simulink model "gantryModel"  (R2025b)
settings: Solver=ode4  StartTime=0.0  StopTime=50  FixedStep=0.01  RelTol=1e-3
values from neighbouring files (symbols this model uses):
  Kda = p(3)    [costFun.m]    (also in plots_tuning.m = gains.Kda(id_gain); tuning.m = Kda(valid))
  Kpa = p(2)    [costFun.m]    (also in plots_tuning.m = gains.Kpa(id_gain); tuning.m = Kpa(valid))
  Kpx = p(1)    [costFun.m]    (also in plots_tuning.m = gains.Kpx(id_gain); tuning.m = Kpx(valid))
libraries: simulink x3, SignalEditorBlockLib x2
settings Model: Creator=David  LastModifiedBy=David

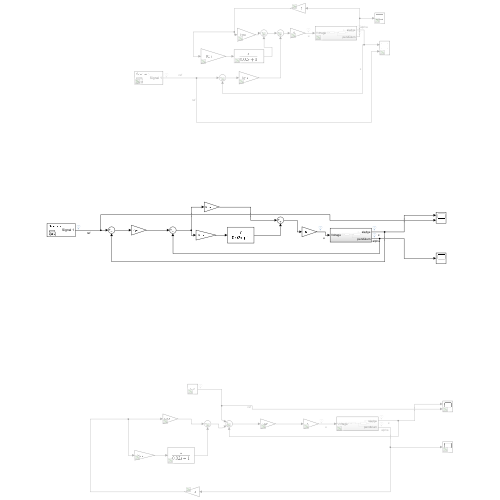
[thumbnail: Simulink's stored preview of the top-level diagram]
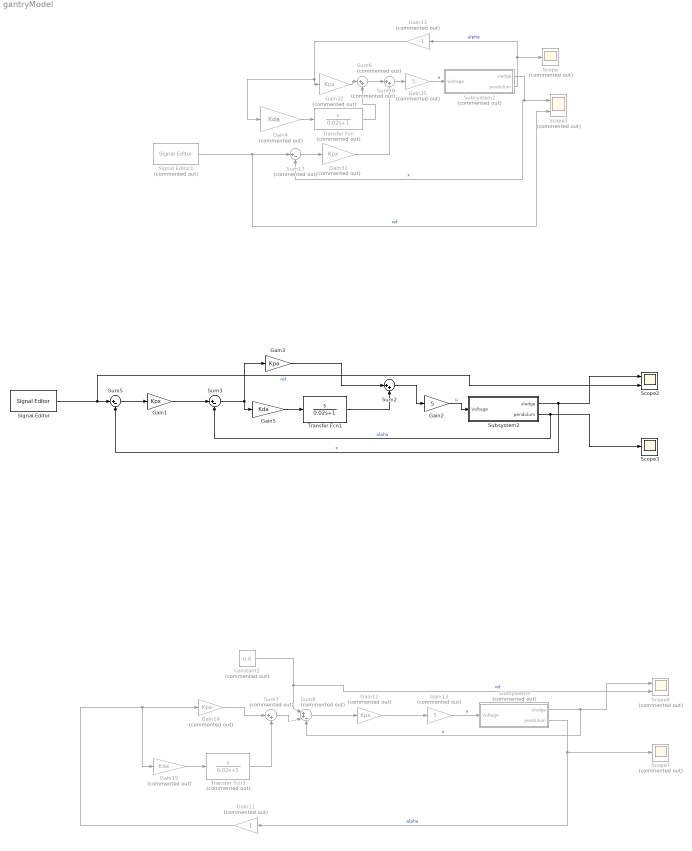
== system gantryModel ==
  Constant2 : Constant  Commented=on  Value=0.8
  Gain1 : Gain  Gain=Kpx
  Gain11 : Gain  Commented=on  Gain=-1
  Gain12 : Gain  Commented=on  Gain=Kpx
  Gain13 : Gain  Commented=on  Gain=5
  Gain14 : Gain  Commented=on  Gain=Kpa
  Gain15 : Gain  Commented=on  Gain=Kda
  Gain2 : Gain  Gain=5
  Gain3 : Gain  Gain=Kpa
  Gain31 : Gain  Commented=on  Gain=Kpx
  Gain32 : Gain  Commented=on  Gain=Kpa
  Gain33 : Gain  Commented=on  Gain=-1
  Gain35 : Gain  Commented=on  Gain=5
  Gain4 : Gain  Commented=on  Gain=Kda
  Gain5 : Gain  Gain=Kda
  Scope : Scope  Commented=on
      settings: ActiveDisplayYMinimum=-4.994410671179125  ActiveDisplayYMaximum=9.4101458764359265
  Scope1 : Scope  Commented=on  NumInputPorts=2
      settings: ActiveDisplayYMinimum=-0.10066051222345068  ActiveDisplayYMaximum=0.90352410472833355
  Scope2 : Scope  NumInputPorts=2
      settings: ActiveDisplayYMinimum=-0.10009126772329788  ActiveDisplayYMaximum=0.90001014085814424  DataLoggingVariableName=ScopeData2
  Scope3 : Scope
      settings: ActiveDisplayYMinimum=-2.552281253947331  ActiveDisplayYMaximum=9.1716981948412979  DataLoggingVariableName=ScopeData3
  Scope6 : Scope  Commented=on  NumInputPorts=2
      settings: ActiveDisplayYMinimum=-0.10533097265407888  ActiveDisplayYMaximum=0.94454271480208  DataLoggingVariableName=ScopeData6
  Scope7 : Scope  Commented=on
      settings: ActiveDisplayYMinimum=-4.9897184342824046  ActiveDisplayYMaximum=9.4373460456385061  DataLoggingVariableName=ScopeData7
  Signal Editor : SignalEditorBlockLib/Signal Editor  FileName=input_tuning.mat  ActiveScenario=Scenario  ActiveSignal=Signal 1  IsBus=off  OutputBusObjectStr=Bus: BusObject  SampleTime=0  ZeroCross=off  OutputAfterFinalValue=Setting to zero  Unit=inherit  PreserveSignalName=on  ApplySigPropsToAllScenarios=on  ApplySigPropsToAllSignals=off  SignalPropertySource=Dialog parameters
  Signal Editor1 : SignalEditorBlockLib/Signal Editor  Commented=on  FileName=input_tuning.mat  ActiveScenario=Scenario  ActiveSignal=Signal 1  IsBus=off  OutputBusObjectStr=Bus: BusObject  SampleTime=0  ZeroCross=off  OutputAfterFinalValue=Setting to zero  Unit=inherit  PreserveSignalName=on  ApplySigPropsToAllScenarios=on  ApplySigPropsToAllSignals=off  SignalPropertySource=Dialog parameters
  Subsystem1 : Subsystem  Commented=on
  Subsystem2 : Subsystem
  Subsystem4 : Subsystem  Commented=on
  Sum16 : Sum  Commented=on  Inputs=|++
  Sum17 : Sum  Commented=on  Inputs=|+-
  Sum2 : Sum  Inputs=|++
  Sum3 : Sum  Inputs=|+-
  Sum5 : Sum  Inputs=|+-
  Sum6 : Sum  Commented=on  Inputs=|++
  Sum7 : Sum  Commented=on  Inputs=|++
  Sum8 : Sum  Commented=on  Inputs=|++-
  Transfer Fcn : TransferFcn  Commented=on  Numerator=[1 0]  Denominator=[0.02 1]
  Transfer Fcn1 : TransferFcn  Numerator=[1 0]  Denominator=[0.02 1]
  Transfer Fcn3 : TransferFcn  Commented=on  Numerator=[1 0]  Denominator=[0.02 1]
  wires:
  Signal Editor1/1 -> Scope1/2, Sum17/1  "ref"
  Gain31/1 -> Sum16/2
  Gain4/1 -> Transfer Fcn/1
  Transfer Fcn/1 -> Sum6/2
  Gain32/1 -> Sum6/1
  Gain35/1 -> Subsystem1/1(Voltage)  "u"
  Sum16/1 -> Gain35/1
  Sum17/1 -> Gain31/1
  Subsystem1/2(pendulum) -> Scope/1, Gain33/1  "alpha"
  Sum6/1 -> Sum16/1
  Subsystem1/1(sledge) -> Sum17/2, Scope1/1  "x"
  Gain33/1 -> Gain4/1, Gain32/1
  Signal Editor/1 -> Scope2/2, Sum5/1  "ref"
  Gain1/1 -> Sum3/1
  Sum3/1 -> Gain3/1, Gain5/1
  Gain3/1 -> Sum2/1
  Gain2/1 -> Subsystem2/1(Voltage)  "u"
  Sum5/1 -> Gain1/1
  Sum2/1 -> Gain2/1
  Transfer Fcn1/1 -> Sum2/2
  Gain5/1 -> Transfer Fcn1/1
  Subsystem2/2(pendulum) -> Sum3/2, Scope3/1  "alpha"
  Subsystem2/1(sledge) -> Scope2/1, Sum5/2  "x"
  Sum7/1 -> Sum8/2
  Constant2/1 -> Scope6/2, Sum8/1  "ref"
  Sum8/1 -> Gain12/1
  Transfer Fcn3/1 -> Sum7/2
  Gain11/1 -> Gain15/1, Gain14/1
  Gain15/1 -> Transfer Fcn3/1
  Gain14/1 -> Sum7/1
  Gain13/1 -> Subsystem4/1(Voltage)  "u"
  Gain12/1 -> Gain13/1
  Subsystem4/2(pendulum) -> Scope7/1, Gain11/1  "alpha"
  Subsystem4/1(sledge) -> Sum8/3, Scope6/1  "x"

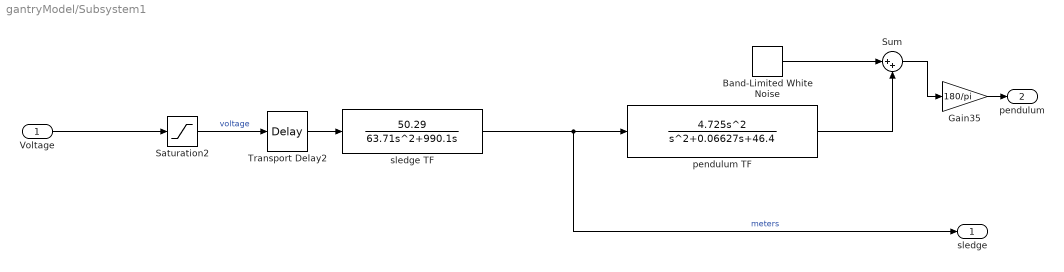
== system gantryModel/Subsystem1 ==
  Voltage : Inport
  Band-Limited White Noise : simulink/Sources/Band-Limited White Noise  Cov=[6e-10]  Ts=0.01  seed=[23341]
  Gain35 : Gain  Gain=180/pi
  Saturation2 : Saturate  UpperLimit=12  LowerLimit=-12
  Sum : Sum  Inputs=|++
  Transport Delay2 : TransportDelay  DelayTime=0.01
  pendulum TF : TransferFcn  Numerator=[4.725 0 0]  Denominator=[1 0.06627 46.4]
  sledge TF : TransferFcn  Numerator=50.29  Denominator="[63.71  990.1 0]"
  sledge : Outport
  pendulum : Outport  Port=2
  wires:
  Saturation2/1 -> Transport Delay2/1  "voltage"
  sledge TF/1 -> pendulum TF/1, sledge/1  "meters"
  Band-Limited White Noise/1 -> Sum/1
  Sum/1 -> Gain35/1
  Voltage/1 -> Saturation2/1
  Transport Delay2/1 -> sledge TF/1
  pendulum TF/1 -> Sum/2
  Gain35/1 -> pendulum/1

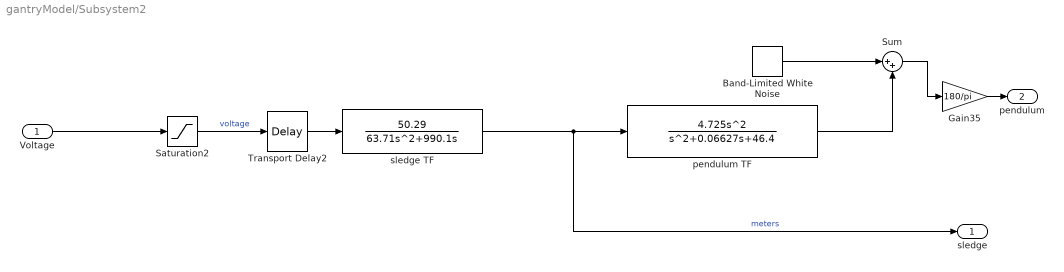
== system gantryModel/Subsystem2 ==
  Voltage : Inport
  Band-Limited White Noise : simulink/Sources/Band-Limited White Noise  Cov=[6e-10]  Ts=0.01  seed=[23341]
  Gain35 : Gain  Gain=180/pi
  Saturation2 : Saturate  UpperLimit=12  LowerLimit=-12
  Sum : Sum  Inputs=|++
  Transport Delay2 : TransportDelay  DelayTime=0.01
  pendulum TF : TransferFcn  Numerator=[4.725 0 0]  Denominator=[1 0.06627 46.4]
  sledge TF : TransferFcn  Numerator=50.29  Denominator="[63.71  990.1 0]"
  sledge : Outport
  pendulum : Outport  Port=2
  wires:
  Saturation2/1 -> Transport Delay2/1  "voltage"
  sledge TF/1 -> pendulum TF/1, sledge/1  "meters"
  Band-Limited White Noise/1 -> Sum/1
  Sum/1 -> Gain35/1
  Voltage/1 -> Saturation2/1
  Transport Delay2/1 -> sledge TF/1
  pendulum TF/1 -> Sum/2
  Gain35/1 -> pendulum/1

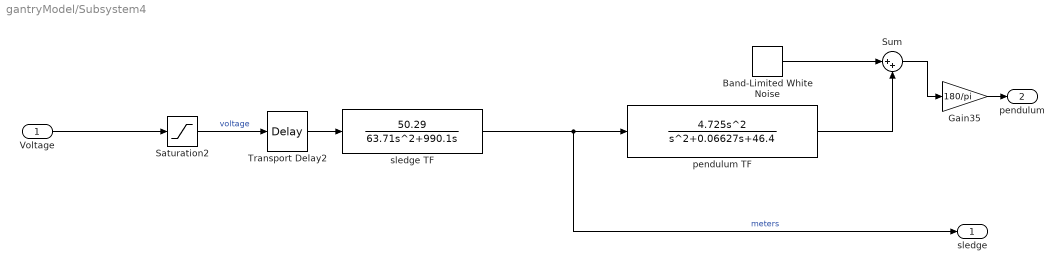
== system gantryModel/Subsystem4 ==
  Voltage : Inport
  Band-Limited White Noise : simulink/Sources/Band-Limited White Noise  Cov=[6e-10]  Ts=0.01  seed=[23341]
  Gain35 : Gain  Gain=180/pi
  Saturation2 : Saturate  UpperLimit=12  LowerLimit=-12
  Sum : Sum  Inputs=|++
  Transport Delay2 : TransportDelay  DelayTime=0.01
  pendulum TF : TransferFcn  Numerator=[4.725 0 0]  Denominator=[1 0.06627 46.4]
  sledge TF : TransferFcn  Numerator=50.29  Denominator="[63.71  990.1 0]"
  sledge : Outport
  pendulum : Outport  Port=2
  wires:
  Saturation2/1 -> Transport Delay2/1  "voltage"
  sledge TF/1 -> pendulum TF/1, sledge/1  "meters"
  Band-Limited White Noise/1 -> Sum/1
  Sum/1 -> Gain35/1
  Voltage/1 -> Saturation2/1
  Transport Delay2/1 -> sledge TF/1
  pendulum TF/1 -> Sum/2
  Gain35/1 -> pendulum/1
